simulink library "csu_stm_simplified_temperature_model_lib"  (R2014b)
settings: Solver=ode45  StartTime=0.0  StopTime=10.0  RelTol=1e-3
libraries: util_info_lib x1
settings Model: Creator=Nilesh  LastModifiedBy=mstewart

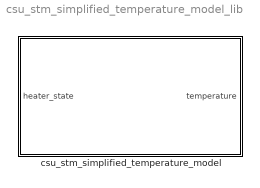
== system csu_stm_simplified_temperature_model_lib ==
  csu_stm_simplified_temperature_model : Subsystem  mask{tc_idx=1, heater_idx=0, initial_temperature=50, min_temperature=-273, max_temperature=273, C1=0.0222, C2=0, C3=0, C4=0, heater_power=0, slope=0, offset=0}
      mask prompts: tc_idx "Temperature Sensor Index"; heater_idx "Heater Index"; initial_temperature "Initial Temperature (C)"; min_temperature "Heater OFF asymptote temperature (C)"; max_temperature "Heater ON asymptote temperature (C)"; C1 "C1: Environmental Heat"; C2 "C2: Dissapative Heat"; C3 "C3: Radiative Heat Terms"; C4 "C4: Conductive Heat Terms"; heater_power "C5: Heater Power"; slope "Conversion to Counts: Slope"; offset "Conversion to Counts: Offset"

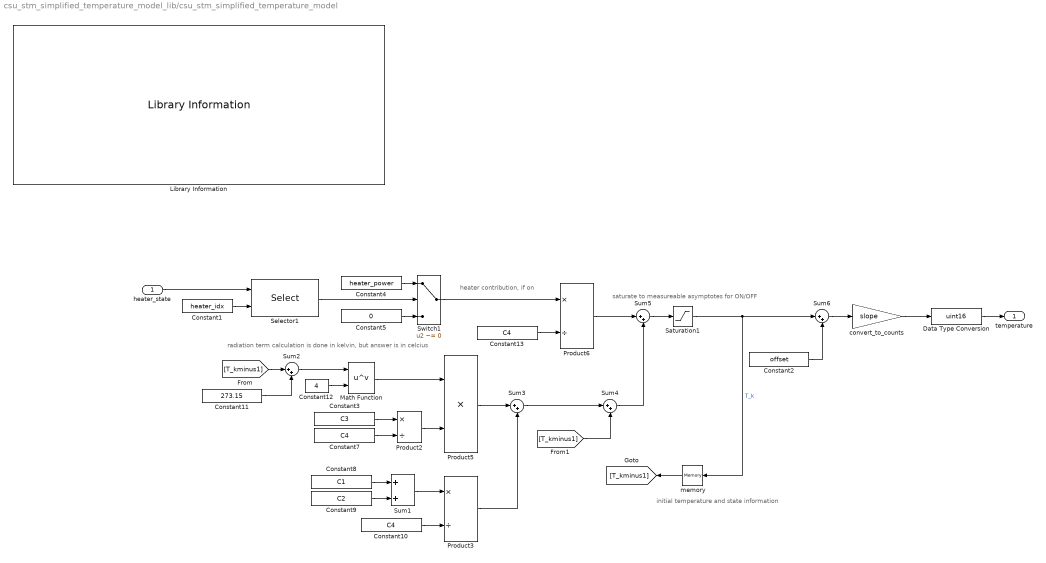
== system csu_stm_simplified_temperature_model_lib/csu_stm_simplified_temperature_model ==
  note: heater contribution, if on
  note: radiation term calculation is done in kelvin, but answer is in celcius
  note: initial temperature and state information
  note: saturate to measureable asymptotes for ON/OFF
  heater_state : Inport
  Constant1 : Constant  Value=heater_idx  OutDataTypeStr=uint8
  Constant10 : Constant  Value=C4  OutDataTypeStr=double
  Constant11 : Constant  Value=273.15  OutDataTypeStr=double
  Constant12 : Constant  Value=4  OutDataTypeStr=double
  Constant13 : Constant  Value=C4  OutDataTypeStr=double
  Constant2 : Constant  Value=offset  OutDataTypeStr=double
  Constant3 : Constant  Value=C3  OutDataTypeStr=double
  Constant4 : Constant  Value=heater_power  OutDataTypeStr=double
  Constant5 : Constant  Value=0  OutDataTypeStr=double
  Constant7 : Constant  Value=C4  OutDataTypeStr=double
  Constant8 : Constant  Value=C1  OutDataTypeStr=double
  Constant9 : Constant  Value=C2  OutDataTypeStr=double
  Data Type Conversion : DataTypeConversion  OutDataTypeStr=uint16
  Library Information : util_info_lib/Library Information  owner='escrane'
  Math Function : Math  Operator=pow  SaturateOnIntegerOverflow=on
  Product2 : Product  Inputs=*/
  Product3 : Product  Inputs=*/
  Product5 : Product
  Product6 : Product  Inputs=*/
  Saturation1 : Saturate  UpperLimit=max_temperature  LowerLimit=min_temperature
  Selector1 : Selector  InputPortWidth=stm_n_heaters  IndexOptions=Index vector (port)  Indices=[1 3]
  Sum1 : Sum
  Sum{2..6} (5 alike) : Sum  Inputs=|++
  Switch1 : Switch  Criteria=u2 ~= 0
  convert_to_counts : Gain  Gain=slope
  memory : Memory  X0=initial_temperature  InheritSampleTime=on
  temperature : Outport
  wires:
  memory/1 -> [T_kminus1]
  Constant1/1 -> Selector1/2
  heater_state/1 -> Selector1/1
  Selector1/1 -> Switch1/2
  Constant4/1 -> Switch1/1
  Constant5/1 -> Switch1/3
  Saturation1/1 -> Sum6/1, memory/1  "T_k"
  Constant3/1 -> Product2/1
  Constant7/1 -> Product2/2
  Constant8/1 -> Sum1/1
  Constant9/1 -> Sum1/2
  Constant10/1 -> Product3/2
  Sum1/1 -> Product3/1
  [T_kminus1] -> Sum2/1
  Constant11/1 -> Sum2/2
  Sum2/1 -> Math Function/1
  Constant12/1 -> Math Function/2
  Product2/1 -> Product5/2
  Math Function/1 -> Product5/1
  Product5/1 -> Sum3/1
  Product3/1 -> Sum3/2
  Sum3/1 -> Sum4/1
  [T_kminus1] -> Sum4/2
  Constant13/1 -> Product6/2
  Switch1/1 -> Product6/1
  Product6/1 -> Sum5/1
  Sum4/1 -> Sum5/2
  Sum5/1 -> Saturation1/1
  Data Type Conversion/1 -> temperature/1
  convert_to_counts/1 -> Data Type Conversion/1
  Constant2/1 -> Sum6/2
  Sum6/1 -> convert_to_counts/1
